simulink model "PNNFT"  (R2020b)
settings: Solver=FixedStepAuto  StartTime=0.0  StopTime=2  FixedStep=Ts  MaxStep=1e-4  RelTol=1e-4  EnableMultiTasking=on
values from neighbouring files (symbols this model uses):
  ECons = 1    [Parameters_Function.m]
  Ts = 5e-4    (= 0.0005)    [Parameters_Function.m]
libraries: powerlib x1
settings Model: Creator=ferna  LastModifiedBy=ferna
settings DataIOCC: ReturnWorkspaceOutputs=off
settings DebuggingCC: ArithmeticOperatorsInVariantConditions=warning
settings SFSimCC: SimUseLocalCustomCode=off  CustomCodeUndefinedFunction=UseInterfaceOnly
settings RTWCC: RTWUseLocalCustomCode=off
settings CodeAppCC: StateflowObjectComments=on

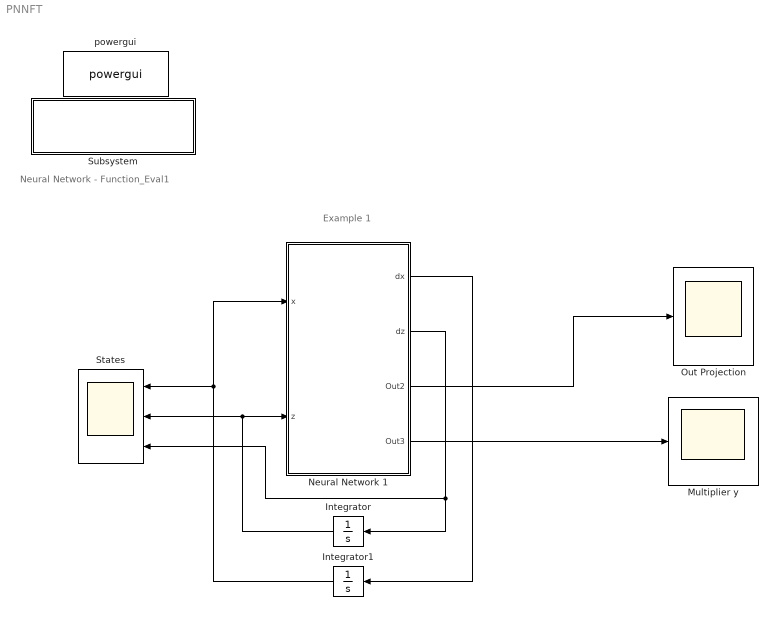
== system PNNFT ==
  note: Example 1
  note: Neural Network - Function_Eval1
  Integrator : Integrator  InitialCondition=-(2.5)*ones(ECons,1)
  Integrator1 : Integrator  InitialCondition=[3,2.5,1]
  Multiplier y : Scope
  Neural Network 1 : MATLAB Function  TreatAsAtomicUnit=on
  Out Projection : Scope
  States : Scope  NumInputPorts=3
  Subsystem : Subsystem
      settings: OpenFcn=open_system('power_new_palette')
      mask Display: disp(sprintf('Open Simscape Power Systems\n(Specialized Technology)\nPalette Library'));
  powergui : powerlib/powergui  Priority=1  SimulationMode=Continuous  SampleTime=Ts  frequency=60  Iterations=50  frequencyindice=60  Pbase=100e6  ErrMax=1e-4  UnitsV=kV  UnitsW=MW  buscounter=0  FunctionMessages=off  echomessages=off  EnableUseOfTLC=off  CurrentSourceSwitches=off  DisableSnubberDevices=off  DisableRonSwitches=off  DisableVfSwitches=off  DisplayEquations=off  AutomaticDiscreteSolvers=off  SolverType=Tustin/Backward Euler (TBE)  Interpol=off  ExternalGateDelay=off  methode=off  Ts=100  x0status=blocks  SPID=off  SwTol=0  HookPort=off  NonlinearTolerance=1e-4  nMaxIteration=100  ContinueOnMaxIteration=off  RestoreLinks=warning  ResistiveCurrentMeasurement=off  Frange=[0:2:500]  Ylog=off  Xlog=on  ShowGrid=off  save=off  variable=ZData  structure=0  ZoomFFT=off  StartTime=0.0  cycles=1  DisplayStyle=1  fundamental=60  FreqAxis=off  MaxFrequency=1000  frequencyindicesteady=1  RmsSteady=1  display=off
  wires:
  Neural Network 1/2(dz) -> Integrator/1, States/3
  Integrator/1 -> Neural Network 1/2(z), States/2
  Neural Network 1/1(dx) -> Integrator1/1
  Integrator1/1 -> States/1, Neural Network 1/1(x)
  Neural Network 1/3(Out2) -> Out Projection/1
  Neural Network 1/4(Out3) -> Multiplier y/1

== system PNNFT/Subsystem ==

== matlab function PNNFT/Neural Network 1 ==
  data: x input; dx output; z input; dz output; Out2 output; Out3 output
function [dx,dz,Out2,Out3] = states(x,z)
%%%%%%%%%%%%%%%%%%%%%%%%%%
%% Calling The Function %%
%%%%%%%%%%%%%%%%%%%%%%%%%%

dx = zeros(length(x),1);
dz = zeros(length(z),1);
Out2 = zeros(length(x),1);
Out3 = zeros(length(x),1);

%Out = zeros(length(Var),1);
%Out2 = zeros(length(x),1);
%Out3 = zeros(length(x),1);

coder.extrinsic('solveSymsN1');
[dx,dz,Out2,Out3] = solveSymsN1(x,z);

%%%%%%%%%%%%%%%%%%%%%%%%%%%%%%%%
% Output Of The Neural Network %
%%%%%%%%%%%%%%%%%%%%%%%%%%%%%%%%
%dx = Out(1:Nvar);
%dz = Out(Nvar+1:end);

end
